simulink model "SAR_ADC_ideal"  (R2018b)
settings: Solver=VariableStepAuto  StartTime=0.0  StopTime=0.001  RelTol=1e-3
values from neighbouring files (symbols this model uses):
  C_mismatch = normrnd(5.75e-14,0,1,32)    [main_SAR_ADC.m]
  fin = 2*pi*200000    (= 1256637.06144)    [main_SAR_ADC.m]
  input_cancel_gain = C_input_cancel./(C_input_cancel + Cp)    [main_SAR_ADC.m]
  R_mismatch = normrnd(200,0,1,64)    [main_SAR_ADC.m]
  Ts = 1/Fs    (= 3.44835710032e-07)    [main_SAR_ADC.m]
  Vos = Avth_pmos*sqrt(W*L)    [main_SAR_ADC.m]
libraries: simulink_extras x51, simulink x1
settings Model: Creator=iamcy  LastModifiedBy=iamcy
settings SolverCC: AlgebraicLoopSolver=LineSearch

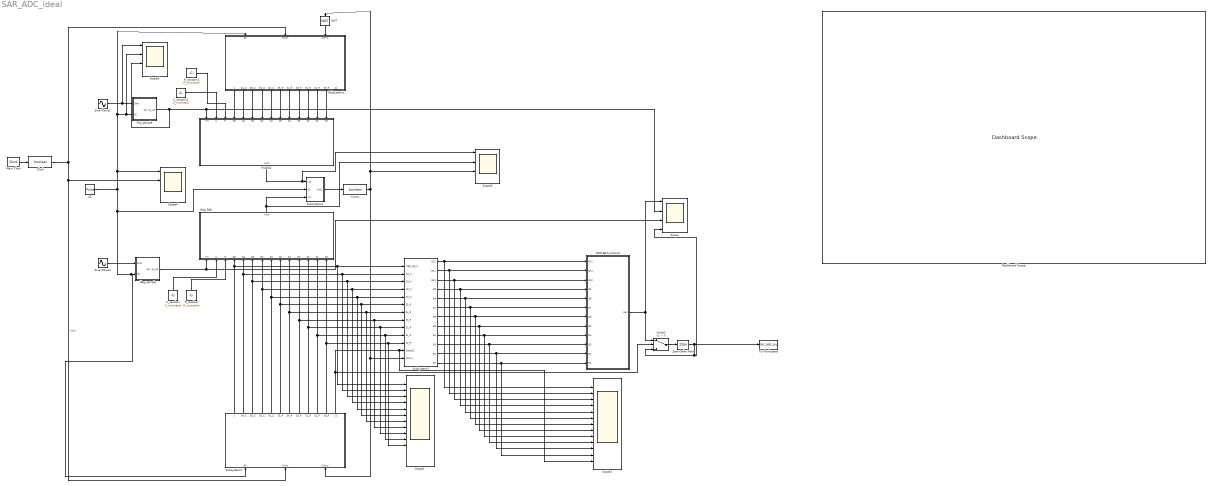
== system SAR_ADC_ideal ==
  C_random : Constant  Value=C_mismatch
  C_random1 : Constant  Value=C_mismatch
  Clock : DataTypeConversion  OutDataTypeStr=boolean
  Comp : DataTypeConversion  OutDataTypeStr=boolean
  Dashboard Scope : DashboardScope  WebBlockId=352
  MATLAB Function2 : MATLAB Function  TreatAsAtomicUnit=on
  Main Clock : simulink_extras/Flip Flops/Clock  period=Tclk
  NOT : Logic  Operator=NOT  IconShape=distinctive  AllPortsSameDT=off  OutDataTypeStr=boolean
  Neg DAC : MATLAB Function  TreatAsAtomicUnit=on
  Neg_sample : Subsystem
  PosDAC : MATLAB Function  TreatAsAtomicUnit=on
  Pos_sample : Subsystem
  R_random : Constant  Value=R_mismatch
  R_random1 : Constant  Value=R_mismatch
  SC : DiscretePulseGenerator  PulseType=Time based  Period=Ts  PulseWidth=100/13
  Scope{,3..5} (4 alike) : Scope  NumInputPorts=4
  Scope1 : Scope  NumInputPorts=13
  Scope2 : Scope  NumInputPorts=13
  Sine Wave2 : Sin  Amplitude=0.5  Frequency=fin  SampleTime=0
  Sine Wave3 : Sin  Amplitude=0.5  Frequency=fin  Phase=pi  SampleTime=0
  Subsystem1 : Subsystem
  Subsystem2 : Subsystem
  Subsystem3 : Subsystem
  Subsystem4 : Subsystem
  Switch : Switch  Criteria=u2 > Threshold
  To Workspace : ToWorkspace  VariableName=sar_adc_out  SampleTime=-1
      settings: Save2DSignal=2-D array (concatenate along first dimension)
  Zero-Order Hold : ZeroOrderHold  SampleTime=Ts
  wires:
  SC/1 -> Subsystem4/2(SC), Subsystem2/1(SC), Neg_sample/2(SC), Subsystem1/1(SC), Scope5/2, Pos_sample/2(SC), Scope4/1
  Neg_sample/1(Sample_out) -> Scope/3, Neg DAC/1(Vin)
  R_random/1 -> Neg DAC/3(R)
  C_random/1 -> Neg DAC/2(C)
  C_random1/1 -> PosDAC/2(C)
  Pos_sample/1(Sample_out) -> Scope5/3, Scope/2, PosDAC/1(Vin)
  R_random1/1 -> PosDAC/3(R)
  PosDAC/1(Vout) -> Scope3/1, Subsystem4/1(Vip)
  Neg DAC/1(Vout) -> Subsystem4/3(Vin), Scope3/2
  Subsystem4/1(Out1) -> Comp/1
  Subsystem1/1(MSB_D5_C) -> PosDAC/4(D5)
  Subsystem1/2(D4_C) -> PosDAC/5(D4)
  Subsystem1/3(D3_C) -> PosDAC/6(D3)
  Subsystem1/4(D2_C) -> PosDAC/7(D2)
  Subsystem1/5(D1_C) -> PosDAC/8(D1)
  Subsystem1/6(S5_R) -> PosDAC/9(S5)
  Subsystem1/7(S4_R) -> PosDAC/10(S4)
  Subsystem1/8(S3_R) -> PosDAC/11(S3)
  Subsystem1/9(S2_R) -> PosDAC/12(S2)
  Subsystem1/10(S1_R) -> PosDAC/13(S1)
  Subsystem1/11(S0_R) -> PosDAC/14(S0)
  Main Clock/1 -> Clock/1
  Clock/1 -> Scope4/2, Subsystem2/2(Clock), Subsystem1/2(Clock)  "clock"
  NOT/1 -> Subsystem1/3(Comp)
  Subsystem2/1(MSB_D5_C) -> Neg DAC/4(D5), Scope1/1, Subsystem3/1(MSB_D5_C)
  Subsystem2/2(D4_C) -> Neg DAC/5(D4), Scope1/2, Subsystem3/2(D4_C)
  Subsystem2/3(D3_C) -> Neg DAC/6(D3), Scope1/3, Subsystem3/3(D3_C)
  Subsystem2/4(D2_C) -> Neg DAC/7(D2), Scope1/4, Subsystem3/4(D2_C)
  Subsystem2/5(D1_C) -> Neg DAC/8(D1), Scope1/5, Subsystem3/5(D1_C)
  Subsystem2/6(S5_R) -> Neg DAC/9(S5), Scope1/6, Subsystem3/6(S5_R)
  Subsystem2/7(S4_R) -> Neg DAC/10(S4), Scope1/7, Subsystem3/7(S4_R)
  Subsystem2/8(S3_R) -> Neg DAC/11(S3), Scope1/8, Subsystem3/8(S3_R)
  Subsystem2/9(S2_R) -> Neg DAC/12(S2), Scope1/9, Subsystem3/9(S2_R)
  Subsystem2/10(S1_R) -> Neg DAC/13(S1), Scope1/10, Subsystem3/10(S1_R)
  Subsystem2/11(S0_R) -> Neg DAC/14(S0), Scope1/11, Subsystem3/11(S0_R)
  Subsystem2/12(State12) -> Switch/2, Scope2/13, Subsystem3/12(State12)
  Subsystem3/1(B12) -> Scope2/1, MATLAB Function2/1(B12)
  Subsystem3/2(B11) -> Scope2/2, MATLAB Function2/2(B11)
  Subsystem3/3(B10) -> Scope2/3, MATLAB Function2/3(B10)
  Subsystem3/4(B9) -> Scope2/4, MATLAB Function2/4(B9)
  Subsystem3/5(B8) -> Scope2/5, MATLAB Function2/5(B8)
  Subsystem3/6(B7) -> Scope2/6, MATLAB Function2/6(B7)
  Subsystem3/7(B6) -> Scope2/7, MATLAB Function2/7(B6)
  Subsystem3/8(B5) -> Scope2/8, MATLAB Function2/8(B5)
  Subsystem3/9(B4) -> Scope2/9, MATLAB Function2/9(B4)
  Subsystem3/10(B3) -> Scope2/10, MATLAB Function2/10(B3)
  Subsystem3/11(B2) -> Scope2/11, MATLAB Function2/11(B2)
  Subsystem3/12(B1) -> Scope2/12, MATLAB Function2/12(B1)
  MATLAB Function2/1(Vout) -> Switch/1, Scope/1
  Comp/1 -> Scope3/3, NOT/1, Subsystem3/13(Comp), Subsystem2/3(Comp)
  Sine Wave2/1 -> Scope5/1, Pos_sample/1(Sine)
  Sine Wave3/1 -> Neg_sample/1(Sine)
  Zero-Order Hold/1 -> Switch/3, Scope/4, To Workspace/1
  Switch/1 -> Zero-Order Hold/1

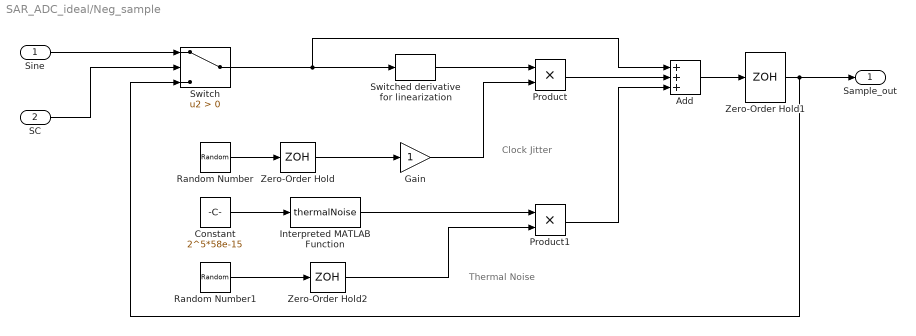
== system SAR_ADC_ideal/Neg_sample ==
  note: Clock Jitter
  note: Thermal Noise
  Sine : Inport
  SC : Inport  Port=2
  Add : Sum  Inputs=3
  Constant : Constant  Value=2^5*58e-15
  Gain : Gain
  Interpreted MATLAB Function : MATLABFcn  MATLABFcn=thermalNoise
  Product : Product
  Product1 : Product
  Random Number : RandomNumber  Variance=30e-12  SampleTime=0.1
  Random Number1 : RandomNumber  Variance=0.01  SampleTime=0.1
  Switch : Switch  Criteria=u2 > Threshold
  Switched derivative for linearization : simulink_extras/Linearization/Switched derivative for linearization  switchVal=1  derivConst=Ts
      settings: SourceProductName=Simulink  SourceProductBaseCode=SL
  Zero-Order Hold : ZeroOrderHold  SampleTime=-1
  Zero-Order Hold1 : ZeroOrderHold  SampleTime=Ts
  Zero-Order Hold2 : ZeroOrderHold  SampleTime=-1
  Sample_out : Outport
  wires:
  Random Number/1 -> Zero-Order Hold/1
  Random Number1/1 -> Zero-Order Hold2/1
  Zero-Order Hold2/1 -> Product1/2
  Switched derivative for linearization/1 -> Product/1
  Interpreted MATLAB Function/1 -> Product1/1
  Product/1 -> Add/2
  Constant/1 -> Interpreted MATLAB Function/1
  Zero-Order Hold1/1 -> Sample_out/1, Switch/3
  Switch/1 -> Switched derivative for linearization/1, Add/1
  Zero-Order Hold/1 -> Gain/1
  Add/1 -> Zero-Order Hold1/1
  Gain/1 -> Product/2
  Product1/1 -> Add/3
  SC/1 -> Switch/2
  Sine/1 -> Switch/1

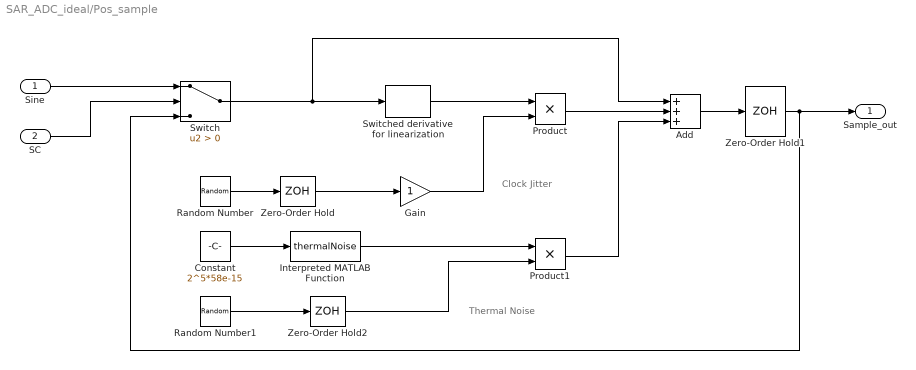
== system SAR_ADC_ideal/Pos_sample ==
  note: Clock Jitter
  note: Thermal Noise
  Sine : Inport
  SC : Inport  Port=2
  Add : Sum  Inputs=3
  Constant : Constant  Value=2^5*58e-15
  Gain : Gain
  Interpreted MATLAB Function : MATLABFcn  MATLABFcn=thermalNoise
  Product : Product
  Product1 : Product
  Random Number : RandomNumber  Variance=30e-12  SampleTime=0.1
  Random Number1 : RandomNumber  Variance=0.01  SampleTime=0.1
  Switch : Switch  Criteria=u2 > Threshold
  Switched derivative for linearization : simulink_extras/Linearization/Switched derivative for linearization  switchVal=1  derivConst=Ts
      settings: SourceProductName=Simulink  SourceProductBaseCode=SL
  Zero-Order Hold : ZeroOrderHold  SampleTime=Ts
  Zero-Order Hold1 : ZeroOrderHold  SampleTime=Ts
  Zero-Order Hold2 : ZeroOrderHold  SampleTime=Ts
  Sample_out : Outport
  wires:
  Random Number/1 -> Zero-Order Hold/1
  Random Number1/1 -> Zero-Order Hold2/1
  Zero-Order Hold2/1 -> Product1/2
  Switched derivative for linearization/1 -> Product/1
  Interpreted MATLAB Function/1 -> Product1/1
  Product/1 -> Add/2
  Constant/1 -> Interpreted MATLAB Function/1
  Zero-Order Hold1/1 -> Sample_out/1, Switch/3
  Switch/1 -> Switched derivative for linearization/1, Add/1
  Zero-Order Hold/1 -> Gain/1
  Add/1 -> Zero-Order Hold1/1
  Gain/1 -> Product/2
  Product1/1 -> Add/3
  SC/1 -> Switch/2
  Sine/1 -> Switch/1

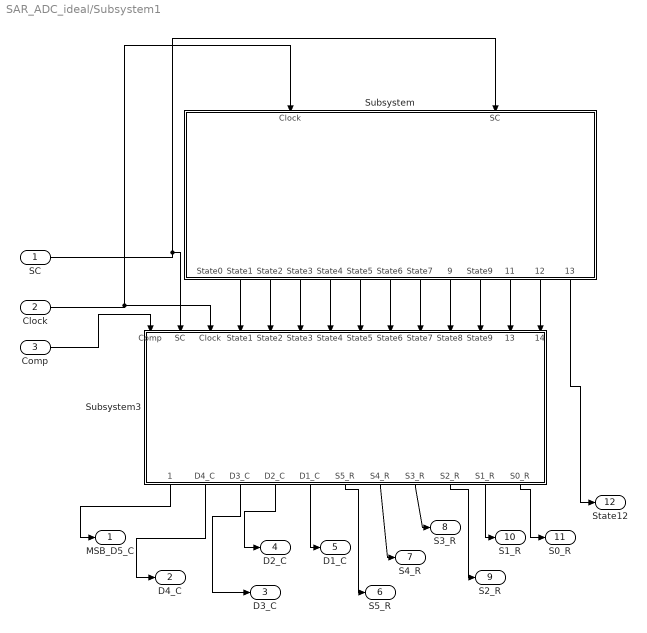
== system SAR_ADC_ideal/Subsystem1 ==
  SC : Inport
  Clock : Inport  Port=2
  Comp : Inport  Port=3
  Subsystem : Subsystem
  Subsystem3 : Subsystem
  MSB_D5_C : Outport
  D4_C : Outport  Port=2
  D3_C : Outport  Port=3
  D2_C : Outport  Port=4
  D1_C : Outport  Port=5
  S5_R : Outport  Port=6
  S4_R : Outport  Port=7
  S3_R : Outport  Port=8
  S2_R : Outport  Port=9
  S1_R : Outport  Port=10
  S0_R : Outport  Port=11
  State12 : Outport  Port=12
  wires:
  SC/1 -> Subsystem3/2(SC), Subsystem/2(SC)
  Subsystem3/9(S2_R) -> S2_R/1
  Subsystem3/7(S4_R) -> S4_R/1
  Subsystem/4(State3) -> Subsystem3/6(State3)
  Subsystem/3(State2) -> Subsystem3/5(State2)
  Subsystem3/6(S5_R) -> S5_R/1
  Subsystem/2(State1) -> Subsystem3/4(State1)
  Subsystem3/5(D1_C) -> D1_C/1
  Clock/1 -> Subsystem/1(Clock), Subsystem3/3(Clock)
  Subsystem/7(State6) -> Subsystem3/9(State6)
  Subsystem/6(State5) -> Subsystem3/8(State5)
  Subsystem/5(State4) -> Subsystem3/7(State4)
  Subsystem3/2(D4_C) -> D4_C/1
  Subsystem/8(State7) -> Subsystem3/10(State7)
  Subsystem3/1(MSB_D5_C) -> MSB_D5_C/1
  Subsystem/12(State11) -> Subsystem3/14(State11)
  Subsystem/10(State9) -> Subsystem3/12(State9)
  Subsystem/11(State10) -> Subsystem3/13(State10)
  Subsystem/9(State08) -> Subsystem3/11(State8)
  Comp/1 -> Subsystem3/1(Comp)
  Subsystem/13(state12) -> State12/1
  Subsystem3/8(S3_R) -> S3_R/1
  Subsystem3/11(S0_R) -> S0_R/1
  Subsystem3/3(D3_C) -> D3_C/1
  Subsystem3/10(S1_R) -> S1_R/1
  Subsystem3/4(D2_C) -> D2_C/1

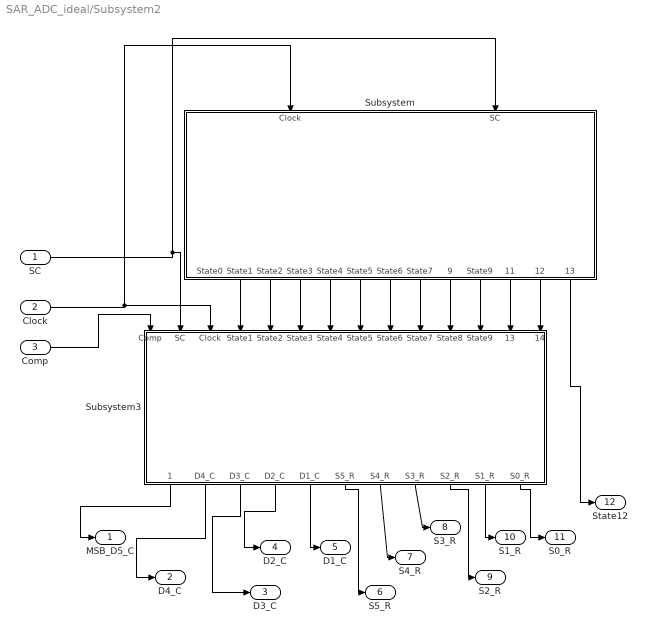
== system SAR_ADC_ideal/Subsystem2 ==
  SC : Inport
  Clock : Inport  Port=2
  Comp : Inport  Port=3
  Subsystem : Subsystem
  Subsystem3 : Subsystem
  MSB_D5_C : Outport
  D4_C : Outport  Port=2
  D3_C : Outport  Port=3
  D2_C : Outport  Port=4
  D1_C : Outport  Port=5
  S5_R : Outport  Port=6
  S4_R : Outport  Port=7
  S3_R : Outport  Port=8
  S2_R : Outport  Port=9
  S1_R : Outport  Port=10
  S0_R : Outport  Port=11
  State12 : Outport  Port=12
  wires:
  SC/1 -> Subsystem3/2(SC), Subsystem/2(SC)
  Subsystem3/9(S2_R) -> S2_R/1
  Subsystem3/7(S4_R) -> S4_R/1
  Subsystem/4(State3) -> Subsystem3/6(State3)
  Subsystem/3(State2) -> Subsystem3/5(State2)
  Subsystem3/6(S5_R) -> S5_R/1
  Subsystem/2(State1) -> Subsystem3/4(State1)
  Subsystem3/5(D1_C) -> D1_C/1
  Clock/1 -> Subsystem/1(Clock), Subsystem3/3(Clock)
  Subsystem/7(State6) -> Subsystem3/9(State6)
  Subsystem/6(State5) -> Subsystem3/8(State5)
  Subsystem/5(State4) -> Subsystem3/7(State4)
  Subsystem3/2(D4_C) -> D4_C/1
  Subsystem/8(State7) -> Subsystem3/10(State7)
  Subsystem3/1(MSB_D5_C) -> MSB_D5_C/1
  Subsystem/12(State11) -> Subsystem3/14(State11)
  Subsystem/10(State9) -> Subsystem3/12(State9)
  Subsystem/11(State10) -> Subsystem3/13(State10)
  Subsystem/9(State08) -> Subsystem3/11(State8)
  Comp/1 -> Subsystem3/1(Comp)
  Subsystem/13(state12) -> State12/1
  Subsystem3/8(S3_R) -> S3_R/1
  Subsystem3/11(S0_R) -> S0_R/1
  Subsystem3/3(D3_C) -> D3_C/1
  Subsystem3/10(S1_R) -> S1_R/1
  Subsystem3/4(D2_C) -> D2_C/1

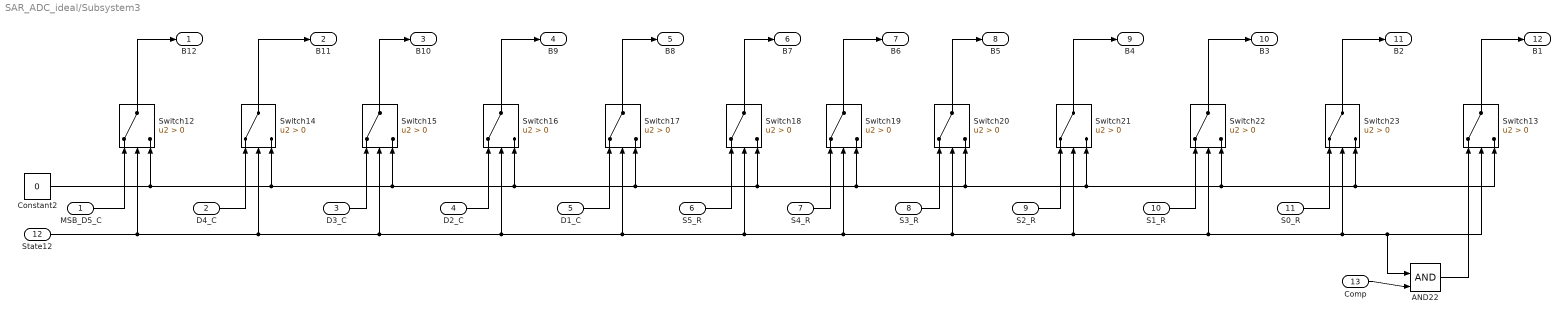
== system SAR_ADC_ideal/Subsystem3 ==
  MSB_D5_C : Inport
  D4_C : Inport  Port=2
  D3_C : Inport  Port=3
  D2_C : Inport  Port=4
  D1_C : Inport  Port=5
  S5_R : Inport  Port=6
  S4_R : Inport  Port=7
  S3_R : Inport  Port=8
  S2_R : Inport  Port=9
  S1_R : Inport  Port=10
  S0_R : Inport  Port=11
  State12 : Inport  Port=12
  Comp : Inport  Port=13
  AND22 : Logic  IconShape=distinctive  AllPortsSameDT=off  OutDataTypeStr=boolean
  Constant2 : Constant  Value=0
  Switch{12..23} (12 alike) : Switch  Criteria=u2 > Threshold
  B12 : Outport
  B11 : Outport  Port=2
  B10 : Outport  Port=3
  B9 : Outport  Port=4
  B8 : Outport  Port=5
  B7 : Outport  Port=6
  B6 : Outport  Port=7
  B5 : Outport  Port=8
  B4 : Outport  Port=9
  B3 : Outport  Port=10
  B2 : Outport  Port=11
  B1 : Outport  Port=12
  wires:
  Constant2/1 -> Switch12/3, Switch13/3, Switch23/3, Switch22/3, Switch21/3, Switch20/3, Switch19/3, Switch18/3, Switch17/3, Switch16/3, Switch15/3, Switch14/3
  Switch22/1 -> B3/1
  Switch17/1 -> B8/1
  Switch12/1 -> B12/1
  Switch14/1 -> B11/1
  Switch18/1 -> B7/1
  Switch16/1 -> B9/1
  Switch15/1 -> B10/1
  Switch23/1 -> B2/1
  Switch20/1 -> B5/1
  Switch21/1 -> B4/1
  Switch19/1 -> B6/1
  Switch13/1 -> B1/1
  State12/1 -> Switch12/2, Switch14/2, Switch15/2, Switch16/2, Switch17/2, Switch19/2, Switch20/2, Switch21/2, Switch22/2, AND22/1, Switch13/2, Switch23/2, Switch18/2
  AND22/1 -> Switch13/1
  Comp/1 -> AND22/2
  S0_R/1 -> Switch23/1
  S1_R/1 -> Switch22/1
  S2_R/1 -> Switch21/1
  S3_R/1 -> Switch20/1
  S4_R/1 -> Switch19/1
  S5_R/1 -> Switch18/1
  D1_C/1 -> Switch17/1
  D2_C/1 -> Switch16/1
  D3_C/1 -> Switch15/1
  D4_C/1 -> Switch14/1
  MSB_D5_C/1 -> Switch12/1

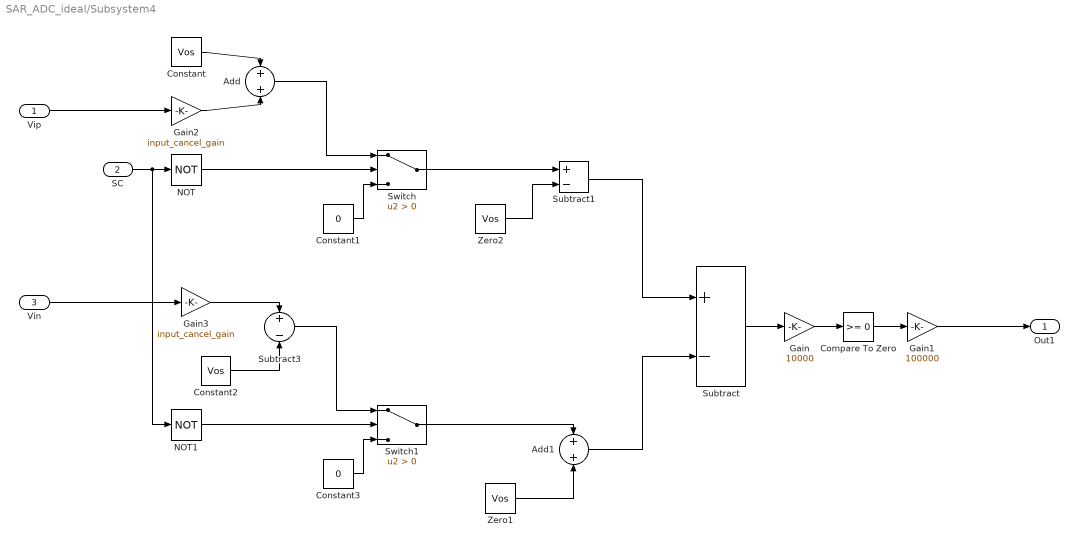
== system SAR_ADC_ideal/Subsystem4 ==
  Vip : Inport
  SC : Inport  Port=2
  Vin : Inport  Port=3
  Add : Sum  Inputs=2
  Add1 : Sum
  Compare To Zero : simulink/Logic and Bit Operations/Compare To Zero  relop=>=  OutDataTypeStr=boolean
  Constant : Constant  Value=Vos
  Constant1 : Constant  Value=0
  Constant2 : Constant  Value=Vos
  Constant3 : Constant  Value=0
  Gain : Gain  Gain=10000
  Gain1 : Gain  Gain=100000
  Gain2 : Gain  Gain=input_cancel_gain
  Gain3 : Gain  Gain=input_cancel_gain
  NOT : Logic  Operator=NOT  IconShape=distinctive  AllPortsSameDT=off  OutDataTypeStr=boolean
  NOT1 : Logic  Operator=NOT  IconShape=distinctive  AllPortsSameDT=off  OutDataTypeStr=boolean
  Subtract : Sum  Inputs=+-
  Subtract1 : Sum  Inputs=+-
  Subtract3 : Sum  Inputs=+-
  Switch : Switch  Criteria=u2 > Threshold
  Switch1 : Switch  Criteria=u2 > Threshold
  Zero1 : Constant  Value=Vos  OutDataTypeStr=Inherit: Inherit via back propagation
  Zero2 : Constant  Value=Vos  OutDataTypeStr=Inherit: Inherit via back propagation
  Out1 : Outport
  wires:
  Compare To Zero/1 -> Gain1/1
  Subtract/1 -> Gain/1
  Subtract1/1 -> Subtract/1
  Gain1/1 -> Out1/1
  Gain/1 -> Compare To Zero/1
  Constant/1 -> Add/1
  Gain2/1 -> Add/2
  Vip/1 -> Gain2/1
  Zero2/1 -> Subtract1/2
  SC/1 -> NOT1/1, NOT/1
  NOT/1 -> Switch/2
  Add/1 -> Switch/1
  Switch/1 -> Subtract1/1
  Constant1/1 -> Switch/3
  Vin/1 -> Gain3/1
  Constant2/1 -> Subtract3/2
  Gain3/1 -> Subtract3/1
  Switch1/1 -> Add1/1
  Zero1/1 -> Add1/2
  NOT1/1 -> Switch1/2
  Constant3/1 -> Switch1/3
  Subtract3/1 -> Switch1/1
  Add1/1 -> Subtract/2

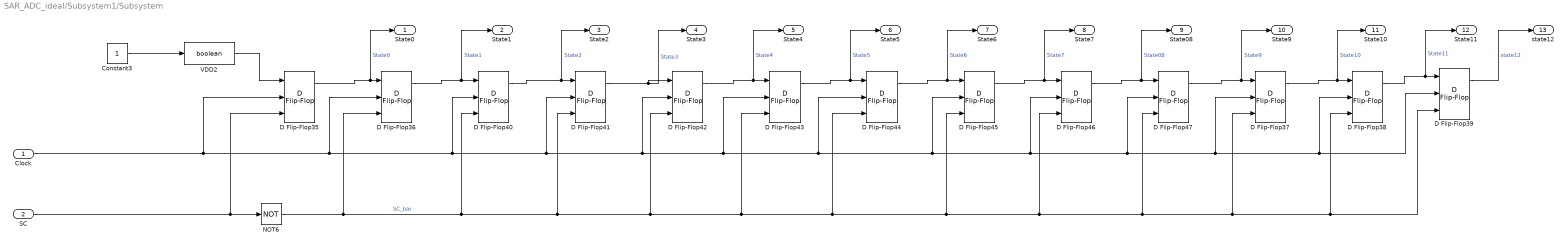
== system SAR_ADC_ideal/Subsystem1/Subsystem ==
  Clock : Inport
  SC : Inport  Port=2
  Constant3 : Constant
  D Flip-Flop{35..47} (13 alike) : simulink_extras/Flip Flops/D Flip-Flop
      settings: SourceProductName=Simulink
  NOT6 : Logic  Operator=NOT  IconShape=distinctive  AllPortsSameDT=off  OutDataTypeStr=boolean
  VDD2 : DataTypeConversion  OutDataTypeStr=boolean
  State0 : Outport
  State1 : Outport  Port=2
  State2 : Outport  Port=3
  State3 : Outport  Port=4
  State4 : Outport  Port=5
  State5 : Outport  Port=6
  State6 : Outport  Port=7
  State7 : Outport  Port=8
  State08 : Outport  Port=9
  State9 : Outport  Port=10
  State10 : Outport  Port=11
  State11 : Outport  Port=12
  state12 : Outport  Port=13
  wires:
  D Flip-Flop43/1 -> State5/1, D Flip-Flop44/1  "State5"
  D Flip-Flop40/1 -> State2/1, D Flip-Flop41/1  "State2"
  D Flip-Flop45/1 -> State7/1, D Flip-Flop46/1  "State7"
  D Flip-Flop38/1 -> State11/1, D Flip-Flop39/1  "State11"
  D Flip-Flop42/1 -> State4/1, D Flip-Flop43/1  "State4"
  D Flip-Flop44/1 -> State6/1, D Flip-Flop45/1  "State6"
  NOT6/1 -> D Flip-Flop42/3, D Flip-Flop44/3, D Flip-Flop46/3, D Flip-Flop38/3, D Flip-Flop39/3, D Flip-Flop37/3, D Flip-Flop47/3, D Flip-Flop45/3, D Flip-Flop43/3, D Flip-Flop41/3, D Flip-Flop40/3, D Flip-Flop36/3  "SC_bar"
  D Flip-Flop36/1 -> State1/1, D Flip-Flop40/1  "State1"
  Clock/1 -> D Flip-Flop36/2, D Flip-Flop41/2, D Flip-Flop42/2, D Flip-Flop43/2, D Flip-Flop44/2, D Flip-Flop45/2, D Flip-Flop46/2, D Flip-Flop38/2, D Flip-Flop39/2, D Flip-Flop37/2, D Flip-Flop47/2, D Flip-Flop40/2, D Flip-Flop35/2
  D Flip-Flop47/1 -> State9/1, D Flip-Flop37/1  "State9"
  Constant3/1 -> VDD2/1
  D Flip-Flop41/1 -> State3/1, D Flip-Flop42/1  "State3"
  D Flip-Flop37/1 -> State10/1, D Flip-Flop38/1  "State10"
  D Flip-Flop35/1 -> State0/1, D Flip-Flop36/1  "State0"
  D Flip-Flop46/1 -> State08/1, D Flip-Flop47/1  "State08"
  SC/1 -> NOT6/1, D Flip-Flop35/3
  VDD2/1 -> D Flip-Flop35/1
  D Flip-Flop39/1 -> state12/1  "state12"

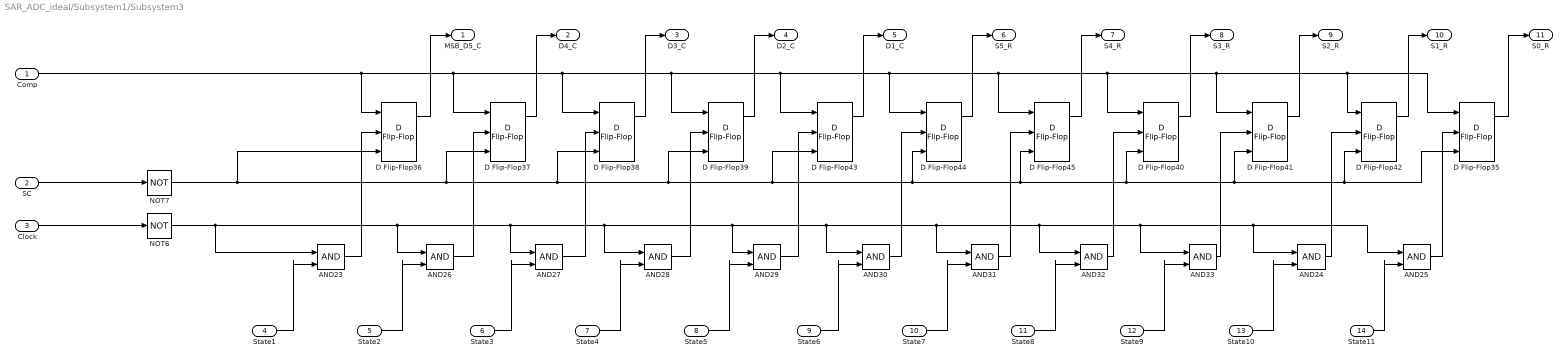
== system SAR_ADC_ideal/Subsystem1/Subsystem3 ==
  Comp : Inport
  SC : Inport  Port=2
  Clock : Inport  Port=3
  State1 : Inport  Port=4
  State2 : Inport  Port=5
  State3 : Inport  Port=6
  State4 : Inport  Port=7
  State5 : Inport  Port=8
  State6 : Inport  Port=9
  State7 : Inport  Port=10
  State8 : Inport  Port=11
  State9 : Inport  Port=12
  State10 : Inport  Port=13
  State11 : Inport  Port=14
  AND{23..33} (11 alike) : Logic  IconShape=distinctive  AllPortsSameDT=off  OutDataTypeStr=boolean
  D Flip-Flop{35..45} (11 alike) : simulink_extras/Flip Flops/D Flip-Flop
      settings: SourceProductName=Simulink
  NOT6 : Logic  Operator=NOT  IconShape=distinctive  AllPortsSameDT=off  OutDataTypeStr=boolean
  NOT7 : Logic  Operator=NOT  IconShape=distinctive  AllPortsSameDT=off  OutDataTypeStr=boolean
  MSB_D5_C : Outport
  D4_C : Outport  Port=2
  D3_C : Outport  Port=3
  D2_C : Outport  Port=4
  D1_C : Outport  Port=5
  S5_R : Outport  Port=6
  S4_R : Outport  Port=7
  S3_R : Outport  Port=8
  S2_R : Outport  Port=9
  S1_R : Outport  Port=10
  S0_R : Outport  Port=11
  wires:
  NOT7/1 -> D Flip-Flop35/3, D Flip-Flop42/3, D Flip-Flop41/3, D Flip-Flop40/3, D Flip-Flop45/3, D Flip-Flop44/3, D Flip-Flop43/3, D Flip-Flop39/3, D Flip-Flop38/3, D Flip-Flop37/3, D Flip-Flop36/3
  D Flip-Flop41/1 -> S2_R/1
  AND23/1 -> D Flip-Flop36/2
  State9/1 -> AND33/2
  Comp/1 -> D Flip-Flop35/1, D Flip-Flop42/1, D Flip-Flop41/1, D Flip-Flop40/1, D Flip-Flop45/1, D Flip-Flop44/1, D Flip-Flop43/1, D Flip-Flop39/1, D Flip-Flop38/1, D Flip-Flop37/1, D Flip-Flop36/1
  D Flip-Flop42/1 -> S1_R/1
  AND27/1 -> D Flip-Flop38/2
  NOT6/1 -> AND25/1, AND24/1, AND33/1, AND32/1, AND31/1, AND30/1, AND29/1, AND28/1, AND27/1, AND26/1, AND23/1
  AND25/1 -> D Flip-Flop35/2
  AND29/1 -> D Flip-Flop43/2
  AND31/1 -> D Flip-Flop45/2
  AND28/1 -> D Flip-Flop39/2
  State1/1 -> AND23/2
  AND33/1 -> D Flip-Flop41/2
  D Flip-Flop45/1 -> S4_R/1
  State5/1 -> AND29/2
  AND26/1 -> D Flip-Flop37/2
  AND24/1 -> D Flip-Flop42/2
  SC/1 -> NOT7/1
  AND32/1 -> D Flip-Flop40/2
  State10/1 -> AND24/2
  AND30/1 -> D Flip-Flop44/2
  D Flip-Flop38/1 -> D3_C/1
  Clock/1 -> NOT6/1
  D Flip-Flop36/1 -> MSB_D5_C/1
  D Flip-Flop37/1 -> D4_C/1
  D Flip-Flop35/1 -> S0_R/1
  D Flip-Flop43/1 -> D1_C/1
  State4/1 -> AND28/2
  State3/1 -> AND27/2
  State2/1 -> AND26/2
  State8/1 -> AND32/2
  D Flip-Flop44/1 -> S5_R/1
  State6/1 -> AND30/2
  State11/1 -> AND25/2
  D Flip-Flop40/1 -> S3_R/1
  State7/1 -> AND31/2
  D Flip-Flop39/1 -> D2_C/1

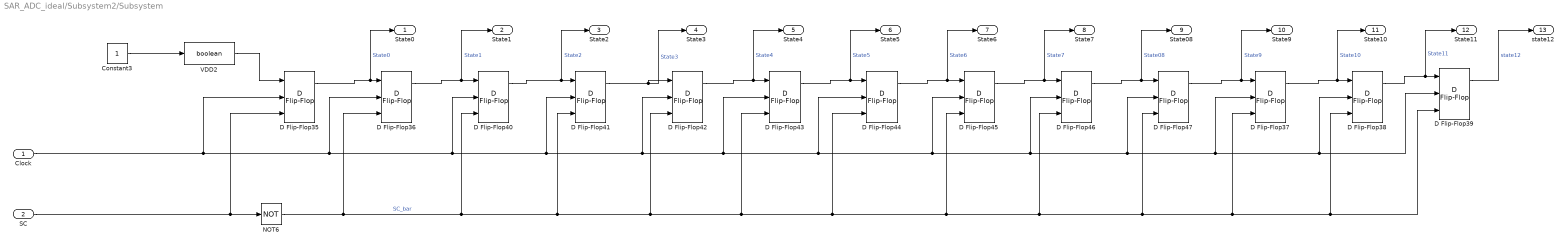
== system SAR_ADC_ideal/Subsystem2/Subsystem ==
  Clock : Inport
  SC : Inport  Port=2
  Constant3 : Constant
  D Flip-Flop{35..47} (13 alike) : simulink_extras/Flip Flops/D Flip-Flop
      settings: SourceProductName=Simulink
  NOT6 : Logic  Operator=NOT  IconShape=distinctive  AllPortsSameDT=off  OutDataTypeStr=boolean
  VDD2 : DataTypeConversion  OutDataTypeStr=boolean
  State0 : Outport
  State1 : Outport  Port=2
  State2 : Outport  Port=3
  State3 : Outport  Port=4
  State4 : Outport  Port=5
  State5 : Outport  Port=6
  State6 : Outport  Port=7
  State7 : Outport  Port=8
  State08 : Outport  Port=9
  State9 : Outport  Port=10
  State10 : Outport  Port=11
  State11 : Outport  Port=12
  state12 : Outport  Port=13
  wires:
  D Flip-Flop43/1 -> State5/1, D Flip-Flop44/1  "State5"
  D Flip-Flop40/1 -> State2/1, D Flip-Flop41/1  "State2"
  D Flip-Flop45/1 -> State7/1, D Flip-Flop46/1  "State7"
  D Flip-Flop38/1 -> State11/1, D Flip-Flop39/1  "State11"
  D Flip-Flop42/1 -> State4/1, D Flip-Flop43/1  "State4"
  D Flip-Flop44/1 -> State6/1, D Flip-Flop45/1  "State6"
  NOT6/1 -> D Flip-Flop42/3, D Flip-Flop44/3, D Flip-Flop46/3, D Flip-Flop38/3, D Flip-Flop39/3, D Flip-Flop37/3, D Flip-Flop47/3, D Flip-Flop45/3, D Flip-Flop43/3, D Flip-Flop41/3, D Flip-Flop40/3, D Flip-Flop36/3  "SC_bar"
  D Flip-Flop36/1 -> State1/1, D Flip-Flop40/1  "State1"
  Clock/1 -> D Flip-Flop36/2, D Flip-Flop41/2, D Flip-Flop42/2, D Flip-Flop43/2, D Flip-Flop44/2, D Flip-Flop45/2, D Flip-Flop46/2, D Flip-Flop38/2, D Flip-Flop39/2, D Flip-Flop37/2, D Flip-Flop47/2, D Flip-Flop40/2, D Flip-Flop35/2
  D Flip-Flop47/1 -> State9/1, D Flip-Flop37/1  "State9"
  Constant3/1 -> VDD2/1
  D Flip-Flop41/1 -> State3/1, D Flip-Flop42/1  "State3"
  D Flip-Flop37/1 -> State10/1, D Flip-Flop38/1  "State10"
  D Flip-Flop35/1 -> State0/1, D Flip-Flop36/1  "State0"
  D Flip-Flop46/1 -> State08/1, D Flip-Flop47/1  "State08"
  SC/1 -> NOT6/1, D Flip-Flop35/3
  VDD2/1 -> D Flip-Flop35/1
  D Flip-Flop39/1 -> state12/1  "state12"

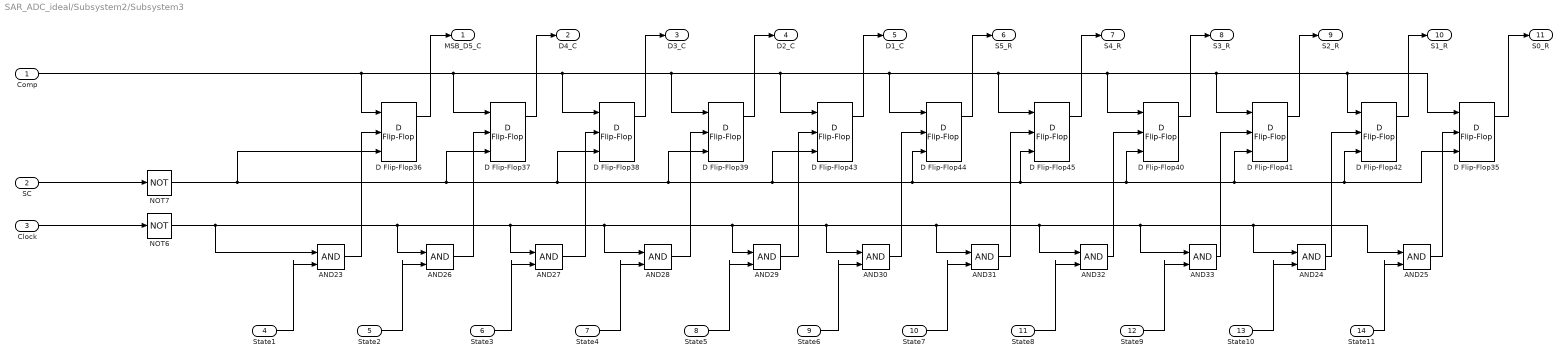
== system SAR_ADC_ideal/Subsystem2/Subsystem3 ==
  Comp : Inport
  SC : Inport  Port=2
  Clock : Inport  Port=3
  State1 : Inport  Port=4
  State2 : Inport  Port=5
  State3 : Inport  Port=6
  State4 : Inport  Port=7
  State5 : Inport  Port=8
  State6 : Inport  Port=9
  State7 : Inport  Port=10
  State8 : Inport  Port=11
  State9 : Inport  Port=12
  State10 : Inport  Port=13
  State11 : Inport  Port=14
  AND{23..33} (11 alike) : Logic  IconShape=distinctive  AllPortsSameDT=off  OutDataTypeStr=boolean
  D Flip-Flop{35..45} (11 alike) : simulink_extras/Flip Flops/D Flip-Flop
      settings: SourceProductName=Simulink
  NOT6 : Logic  Operator=NOT  IconShape=distinctive  AllPortsSameDT=off  OutDataTypeStr=boolean
  NOT7 : Logic  Operator=NOT  IconShape=distinctive  AllPortsSameDT=off  OutDataTypeStr=boolean
  MSB_D5_C : Outport
  D4_C : Outport  Port=2
  D3_C : Outport  Port=3
  D2_C : Outport  Port=4
  D1_C : Outport  Port=5
  S5_R : Outport  Port=6
  S4_R : Outport  Port=7
  S3_R : Outport  Port=8
  S2_R : Outport  Port=9
  S1_R : Outport  Port=10
  S0_R : Outport  Port=11
  wires:
  NOT7/1 -> D Flip-Flop35/3, D Flip-Flop42/3, D Flip-Flop41/3, D Flip-Flop40/3, D Flip-Flop45/3, D Flip-Flop44/3, D Flip-Flop43/3, D Flip-Flop39/3, D Flip-Flop38/3, D Flip-Flop37/3, D Flip-Flop36/3
  D Flip-Flop41/1 -> S2_R/1
  AND23/1 -> D Flip-Flop36/2
  State9/1 -> AND33/2
  Comp/1 -> D Flip-Flop35/1, D Flip-Flop42/1, D Flip-Flop41/1, D Flip-Flop40/1, D Flip-Flop45/1, D Flip-Flop44/1, D Flip-Flop43/1, D Flip-Flop39/1, D Flip-Flop38/1, D Flip-Flop37/1, D Flip-Flop36/1
  D Flip-Flop42/1 -> S1_R/1
  AND27/1 -> D Flip-Flop38/2
  NOT6/1 -> AND25/1, AND24/1, AND33/1, AND32/1, AND31/1, AND30/1, AND29/1, AND28/1, AND27/1, AND26/1, AND23/1
  AND25/1 -> D Flip-Flop35/2
  AND29/1 -> D Flip-Flop43/2
  AND31/1 -> D Flip-Flop45/2
  AND28/1 -> D Flip-Flop39/2
  State1/1 -> AND23/2
  AND33/1 -> D Flip-Flop41/2
  D Flip-Flop45/1 -> S4_R/1
  State5/1 -> AND29/2
  AND26/1 -> D Flip-Flop37/2
  AND24/1 -> D Flip-Flop42/2
  SC/1 -> NOT7/1
  AND32/1 -> D Flip-Flop40/2
  State10/1 -> AND24/2
  AND30/1 -> D Flip-Flop44/2
  D Flip-Flop38/1 -> D3_C/1
  Clock/1 -> NOT6/1
  D Flip-Flop36/1 -> MSB_D5_C/1
  D Flip-Flop37/1 -> D4_C/1
  D Flip-Flop35/1 -> S0_R/1
  D Flip-Flop43/1 -> D1_C/1
  State4/1 -> AND28/2
  State3/1 -> AND27/2
  State2/1 -> AND26/2
  State8/1 -> AND32/2
  D Flip-Flop44/1 -> S5_R/1
  State6/1 -> AND30/2
  State11/1 -> AND25/2
  D Flip-Flop40/1 -> S3_R/1
  State7/1 -> AND31/2
  D Flip-Flop39/1 -> D2_C/1

== matlab function SAR_ADC_ideal/PosDAC ==
  data: Vin input; C input; R input; Vout output; D5 input; D4 input; D3 input; D2 input; D1 input; S5 input; S4 input; S3 input; S2 input; S1 input; S0 input
function Vout  = RC_DAC(Vin,C,R,D5,D4,D3,D2,D1,S5,S4,S3,S2,S1,S0)
%%%%%%%%%%%%%%%%%%%%%%%%%%%%%%%%%%%%%%%%%%%%%%%%%%%%%%
% 2018/12/3
% Purpose:  This file is to module R C DAC
%          
%   Copyright (c) 2018 by Shanshan Xie
%   for SAR ADC project in ADC course
%%%%%%%%%%%%%%%%%%%%%%%%%%%%%%%%%%%%%%%%%%%%%%%%%%%%%%


W = 0.13;
L=0.065;
Cp = W*L*6e-15;

N_CDAC = 5;
N_RDAC = 6;
% N_DAC = N_CDAC+N_RDAC;

% Cu = 57.596e-15;
% Ru = 200;

Vref = 1;

%% Switch for C DAC
%  D5 D4 D3 D2 D1
D = [D5 D4 D3 D2 D1]; 

%% Switch for R DAC
thisSwitch = S5*2^5 + S4*2^4 + S3*2^3 + S2*2^2 + S1*2^1 + S0*2^0;


%% Generate C, R with mismatch 32 number of C and 64 number of R
% C = normrnd(1,sigma_C,[1,(2^5)]);
% C = normrnd(1,sigma_C,[1,(2^N_CDAC)]);

% R = normrnd(1,sigma_R,[1,(2^N_RDAC)]);
% R = normrnd(1,sigma_R,[1,(2^N_RDAC)]);


C_binary = C(1);
N_b = 2;

%% generate binary Cap value for cap DAC
for i = 1:N_CDAC-1
    C_binary = [sum(C(N_b:(N_b+N_b-1))), C_binary];
    N_b = N_b*2;
end
C0 = C(2^N_CDAC);
Ctotal = sum(C);

%% Generate Thermometer R DAC

R_seq = zeros(1,length(R));
for i=2:length(R)
   R_seq(:,i) = [sum(R(1:i-1))];

end

% R_seq = fliplr(R_seq);
% R_seq = repmat(R_seq(1:2^N_RDAC),2^N_RDAC,1);

Rtotal = sum(R);

%% Generate Cap voltage
CD = zeros(1,5);
for i = 1:5
   CD(:,i) = C_binary(i)*D(i);
end

Vout_cap = (sum(CD)*Vref) / (Ctotal+Cp);

%% Generate Resistor Voltage
Vout_res = (Vref * C0 * R_seq(thisSwitch+1)) / (Rtotal * (Cp+Ctotal));

Vout = Vout_cap + Vout_res + Vin;

== matlab function SAR_ADC_ideal/Neg DAC ==
  data: Vin input; C input; R input; Vout output; D5 input; D4 input; D3 input; D2 input; D1 input; S5 input; S4 input; S3 input; S2 input; S1 input; S0 input
function Vout  = RC_DAC(Vin,C,R,D5,D4,D3,D2,D1,S5,S4,S3,S2,S1,S0)
%%%%%%%%%%%%%%%%%%%%%%%%%%%%%%%%%%%%%%%%%%%%%%%%%%%%%%
% 2018/12/3
% Purpose:  This file is to module R C DAC
%          
%   Copyright (c) 2018 by Shanshan Xie
%   for SAR ADC project in ADC course
%%%%%%%%%%%%%%%%%%%%%%%%%%%%%%%%%%%%%%%%%%%%%%%%%%%%%%
W = 0.13;
L=0.065;
Cp = W*L*6e-15;

N_CDAC = 5;
N_RDAC = 6;
% N_DAC = N_CDAC+N_RDAC;

% Cu = 57.596e-15;
% Ru = 200;

Vref = 1;

%% Switch for C DAC
%  D5 D4 D3 D2 D1
D = [D5 D4 D3 D2 D1]; 

%% Switch for R DAC
thisSwitch = S5*2^5 + S4*2^4 + S3*2^3 + S2*2^2 + S1*2^1 + S0*2^0;


%% Generate C, R with mismatch 32 number of C and 64 number of R
% C = normrnd(1,sigma_C,[1,(2^5)]);
% C = normrnd(1,sigma_C,[1,(2^N_CDAC)]);

% R = normrnd(1,sigma_R,[1,(2^N_RDAC)]);
% R = normrnd(1,sigma_R,[1,(2^N_RDAC)]);


C_binary = C(1);
N_b = 2;

%% generate binary Cap value for cap DAC
for i = 1:N_CDAC-1
    C_binary = [sum(C(N_b:(N_b+N_b-1))), C_binary];
    N_b = N_b*2;
end
C0 = C(2^N_CDAC);
Ctotal = sum(C);

%% Generate Thermometer R DAC

R_seq = zeros(1,length(R));
for i=2:length(R)
   R_seq(:,i) = [sum(R(1:i-1))];

end

% R_seq = fliplr(R_seq);
% R_seq = repmat(R_seq(1:2^N_RDAC),2^N_RDAC,1);

Rtotal = sum(R);

%% Generate Cap voltage
CD = zeros(1,5);
for i = 1:5
   CD(:,i) = C_binary(i)*D(i);
end

Vout_cap = (sum(CD)*Vref) / (Ctotal+Cp);

%% Generate Resistor Voltage
Vout_res = (Vref * C0 * R_seq(thisSwitch+1)) / (Rtotal * (Cp+Ctotal));

Vout = Vout_cap + Vout_res + Vin;

== matlab function SAR_ADC_ideal/MATLAB Function2 ==
  data: B12 input; Vout output; B11 input; B10 input; B9 input; B8 input; B7 input; B6 input; B5 input; B4 input; B3 input; B2 input; B1 input
function Vout  = ideal_outputDAC(B12,B11,B10,B9,B8,B7,B6,B5,B4,B3,B2,B1)

Vref = 1;
Vout_code = B12*2^11+B11*2^10+B10*2^9+B9*2^8+B8*2^7+B7*2^6+B6*2^5+B5*2^4+B4*2^3+B3*2^2+B2*2^1+B1*2^0;

Vout=(Vout_code*Vref)/2^12;
